simulink model "UAV_Animation"  (R2014a)
settings: Solver=ode45  StartTime=0.0  StopTime=10000  RelTol=1e-3
undefined symbols (not defined in the file or in its folder): drawUAV
libraries: simulink x6
settings Model: Creator=beard  LastModifiedBy=danst_000
settings DataIOCC: SignalLoggingSaveFormat=ModelDataLogs
settings OptimizationCC: ExpressionDepthLimit=2147483647  InitFltsAndDblsToZero=on
settings DebuggingCC: UnderspecifiedInitializationDetection=Classic  FcnCallInpInsideContextMsg=UseLocalSettings  StateNameClashWarn=warning
settings GRTTargetCC: CombineOutputUpdateFcns=off  GRTInterface=on

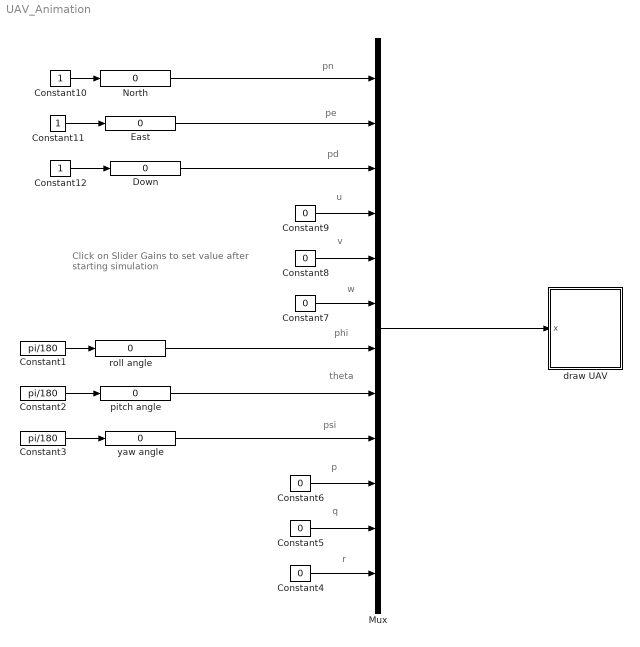
== system UAV_Animation ==
  note: pn
  note: pe
  note: pd
  note: phi
  note: theta
  note: psi
  note: p
  note: q
  note: r
  note: u
  note: v
  note: w
  note: Click on Slider Gains to set value
      | after starting simulation
  Constant1 : Constant  Value=pi/180
  Constant10 : Constant
  Constant11 : Constant
  Constant12 : Constant
  Constant2 : Constant  Value=pi/180
  Constant3 : Constant  Value=pi/180
  Constant{4..9} (6 alike) : Constant  Value=0
  Down : simulink/Math Operations/Slider Gain  low=-10  gain=0  high=10
  East : simulink/Math Operations/Slider Gain  low=-10  gain=0  high=10
  Mux : Mux  Inputs=12
  North : simulink/Math Operations/Slider Gain  low=-10  gain=0  high=10
  draw UAV : Subsystem
      mask init:
      | % define vertices  
      | V = [...
      |         5, 0, 0; ...
      |         3, 1, -1; ...
      |         3, -1, -1; ...
      |         3, -1, 1; ...
      |         3, 1, 1; ...
      |         -4, 0, 0; ...
      |         1, 4, 0; ...
      |         -1, 4, 0; ...
      |         -1, -4, 0; ...
      |         1, -4, 0; ...
      |         -3, 2, 0; ...
      |         -4, 2, 0; ...
      |         -4, -2, 0; ...
      |         -3, -2, 0; ...
      |         -3, 0, 0; ...
      |         -4, 0, -2; ...
      |    ];
      | 
      | % define faces as a list of vertices numbered above
      | F = [...
      |         1, 2, 3, 1; ...
      |         1, 3, 4, 1; ...
      |         1, 4, 5, 1; ...
      |         1, 2, 5, 1; ...
      |         2, 3, 6, 2; ...
      |         3, 4, 6, 3; ...
      |         4, 5, 6, 4; ...
      |         2, 5, 6, 2; ...
      |         7, 8, 9, 10; ...
      |         11, 12, 13, 14; ...
      |         6, 15, 16, 6; ...
      |     ];
      | 
      | 
      | % define colors for each face    
      |   myred = [1, 0, 0];
      |   mygreen = [0, 1, 0];
      |   myblue = [0, 0, 1];
      |   myyellow = [1, 1, 0];
      |   mycyan = [0, 1, 1];
      | 
      |   patchcolors = [...
      |     myred;...    
      |     mygreen;...  
      |     myblue;...   
      |     myyellow;... 
      |     myred;...    
      |     mygreen;...  
      |     myblue;...   
      |     myyellow;... 
      |     mycyan;...   
      |     mycyan;...   
      |     mycyan;...
      |     ];
      mask Display: image(imread('tv.jpg'))
  pitch angle : simulink/Math Operations/Slider Gain  low=-180  gain=0  high=180
  roll angle : simulink/Math Operations/Slider Gain  low=-180  gain=0  high=180
  "yaw angle " : simulink/Math Operations/Slider Gain  low=-180  gain=0  high=180
  wires:
  Mux/1 -> draw UAV/1(x)
  roll angle/1 -> Mux/7
  Constant1/1 -> roll angle/1
  pitch angle/1 -> Mux/8
  Constant2/1 -> pitch angle/1
  "yaw angle "/1 -> Mux/9
  Constant3/1 -> "yaw angle "/1
  Constant4/1 -> Mux/12
  Constant5/1 -> Mux/11
  Constant6/1 -> Mux/10
  Constant7/1 -> Mux/6
  Constant8/1 -> Mux/5
  Constant9/1 -> Mux/4
  North/1 -> Mux/1
  Constant10/1 -> North/1
  East/1 -> Mux/2
  Constant11/1 -> East/1
  Down/1 -> Mux/3
  Constant12/1 -> Down/1

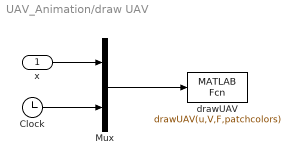
== system UAV_Animation/draw UAV ==
  x : Inport
  Clock : Clock
  Mux : Mux  Inputs=2
  drawUAV : MATLABFcn  MATLABFcn=drawUAV(u,V,F,patchcolors)  OutputDimensions=0  SampleTime=0.1
  wires:
  Mux/1 -> drawUAV/1
  x/1 -> Mux/1
  Clock/1 -> Mux/2
